simulink model "CHEM_FULL_BENCHMARK"  (R2019a)
settings: Solver=FixedStepAuto  StartTime=0.0  StopTime=app.SimuTime  FixedStep=Te  RelTol=1e-3  EnableMultiTasking=on
values from neighbouring files (symbols this model uses):
  A1 = 0.0154    [INIT_FULL.m]    (also in run.m)
  A2 = 0.0154    [INIT_FULL.m]    (also in run.m)
  app = interface    [INIT_FULL.m]    (also in run.m)
  Cvb = 1.5938*1e-4    (= 0.00015938)    [INIT_FULL.m]    (also in run.m)
  Cvo = 1.59640*1e-4    (= 0.00015964)    [INIT_FULL.m]    (also in run.m)
  g = 9.81    [INIT_FULL.m]    (also in run.m)
  h1c = 0.5    [INIT_FULL.m]    (also in run.m)
  h1c_0 = 0    [INIT_FULL.m]    (also in run.m)
  h1max = 0.6    [INIT_FULL.m]    (also in run.m)
  h2c_0 = 0    [INIT_FULL.m]    (also in Variables_Update.m = app.InitialwaterlevelinT206EditField.Value; run.m)
  h2c_max = 0.11    [INIT_FULL.m]    (also in run.m)
  h2c_min = 0.09    [INIT_FULL.m]    (also in run.m)
  h2max = 0.6    [INIT_FULL.m]    (also in run.m)
  Ki = 5*1e-6    (= 5e-06)    [INIT_FULL.m]    (also in run.m)
  Kp = 1e-3    (= 0.001)    [INIT_FULL.m]    (also in run.m)
  Patm = 101325    [INIT_FULL.m]    (also in run.m)
  Qf1 = 1e-4    (= 0.0001)    [INIT_FULL.m]    (also in Variables_Update.m = app.FlowleakfromT1m3sEditField.Value; run.m)
  Qf2 = 1e-4    (= 0.0001)    [INIT_FULL.m]    (also in Variables_Update.m = app.FlowleakfromT2m3sEditField.Value; run.m)
  Qof1 = 1e-4    (= 0.0001)    [INIT_FULL.m]    (also in Variables_Update.m = app.OverflowrateinT1m3sEditField.Value; run.m)
  Qpmax = 1e-2    (= 0.01)    [INIT_FULL.m]    (also in run.m)
  rate_noise_mQp = 0.01*1e-5    (= 1e-07)    [INIT_FULL.m]    (also in run.m)
  rate_noise_mUp = 0.01*1e-5    (= 1e-07)    [INIT_FULL.m]    (also in run.m)
  rate_noise_my1 = 0.5*0.001    (= 0.0005)    [INIT_FULL.m]    (also in run.m)
  rate_noise_my2 = 0.3*0.001    (= 0.0003)    [INIT_FULL.m]    (also in run.m)
  ro = 1000    [INIT_FULL.m]    (also in run.m)
  seed = randi(10000000)    [INIT_FULL.m]    (also in run.m)
  Te = 1    [INIT_FULL.m]    (also in run.m)
  yo = 0    [INIT_FULL.m]    (also in run.m)
(part 1 of 12)
settings Model: Creator=upcnet  LastModifiedBy=etse
settings DataIOCC: LimitDataPoints=on  SaveFormat=Array  ReturnWorkspaceOutputs=off  SignalLoggingName=sigsOut
settings OptimizationCC: BlockReduction=off  BooleanDataType=off  LifeSpan=inf
settings DebuggingCC: AlgebraicLoopMsg=none  SaveWithParameterizedLinksMsg=none  UnderspecifiedInitializationDetection=Classic  MergeDetectMultiDrivingBlocksExec=none  SignalResolutionControl=TryResolveAllWithWarning  MultiTaskDSMMsg=warning  MultiTaskCondExecSysMsg=none  AllowSymbolicDim=off  PregeneratedLibrarySubsystemCodeDiagnostic=none  SFUnexpectedBacktrackingDiag=warning  SFNoUnconditionalDefaultTransitionDiag=warning  SFExecutionAtInitializationDiag=none  ArithmeticOperatorsInVariantConditions=warning
settings HardwareCC: ProdBitPerPointer=32  ProdBitPerSizeT=32  ProdBitPerPtrDiffT=32  ProdLargestAtomicFloat=None  ProdIntDivRoundTo=Undefined  ProdEndianess=Unspecified  ProdWordSize=32  ProdHWDeviceType=32-bit Generic  TargetUnknown=on
settings ModelReferenceCC: PropagateSignalLabelsOutOfModel=off
settings SFSimCC: SimUseLocalCustomCode=off
settings RTWCC: RTWUseLocalCustomCode=off
settings CodeAppCC: StateflowObjectComments=on
settings GRTTargetCC: TargetLangStandard=C89/C90 (ANSI)  CombineOutputUpdateFcns=off  GRTInterface=on
settings ConfigComp: CovMetricSettings=dw  CovHtmlReporting=on  CovSaveCumulativeToWorkspaceVar=on  CovSaveSingleToWorkspaceVar=on  CovExternalEMLEnable=off

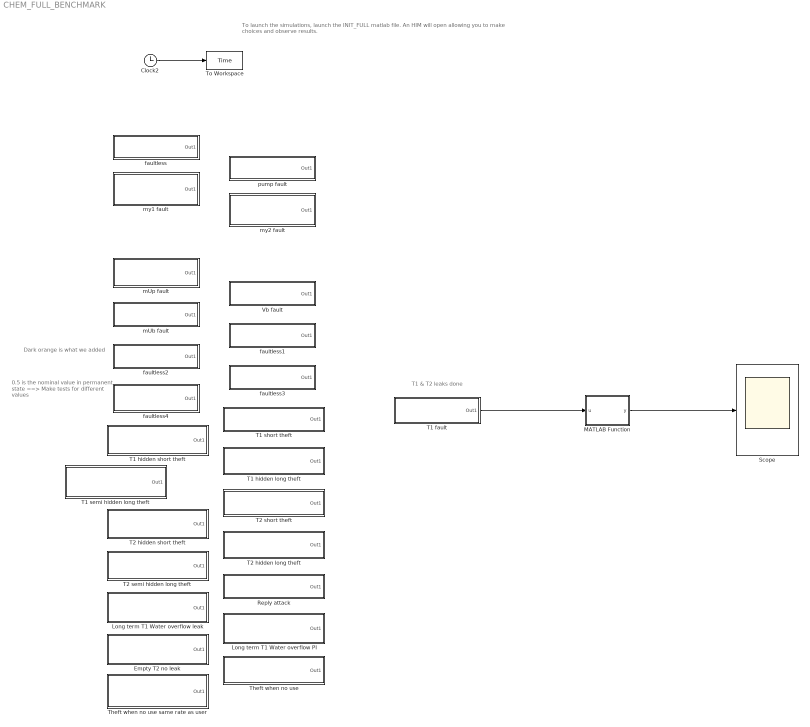
== system CHEM_FULL_BENCHMARK ==
  note: T1 & T2 leaks done
  note: To launch the simulations, launch the INIT_FULL matlab file. An HIM will open allowing you to make choices and observe results.
  note: 0.5 is the nominal value
      | in permanent  state
      | ==> Make tests for different values
  note: Dark orange is what we added
  Clock2 : Clock
  Empty T2 no leak : Subsystem
      mask Display: disp('25) Attack 12\nEmptying T2 without leak')
  Long term T1 Water overflow PI : Subsystem
      mask Display: disp('24) Attack 11\nLong term T1 Water overflow\nWith PI pass by')
  Long term T1 Water overflow leak : Subsystem
      mask Display: disp('23) Attack 10\nLong term T1 Water overflow\nWith simulated leak')
  MATLAB Function : MATLAB Function  TreatAsAtomicUnit=on
  Reply attack : Subsystem
      mask Display: disp('22) Attack 9\nReplay attack')
  Scope : Scope
  T1 fault : Subsystem
      mask Display: disp('5) Fault 4\nTank T1 leak fault: Qf1')
  T1 hidden long theft : Subsystem
      mask Display: disp('16) Attack 3\nLong-term water theft of T1\n without any change of my1')
  T1 hidden short theft : Subsystem
      mask Display: disp('15) Attack 2\nShort-term water theft of T1\n without any change of my1')
  T1 semi hidden long theft : Subsystem
      mask Display: disp('17) Attack 4\nLong-term water theft of T1\nwith a small change of my1')
  T1 short theft : Subsystem
      mask Display: disp('14) Attack 1\nShort-term water theft of T1')
  T2 hidden long theft : Subsystem
      mask Display: disp('20) Attack 7\nLong-term water theft of T2\n without any change of my2')
  T2 hidden short theft : Subsystem
      mask Display: disp('19) Attack 6\nShort-term water theft of T2\n without any change of my2')
  T2 semi hidden long theft : Subsystem
      mask Display: disp('21) Attack 8\nLong-term water theft of T2\n with a small change of my2')
  T2 short theft : Subsystem
      mask Display: disp('18) Attack 5\nShort-term water theft of T2')
  Theft when no use : Subsystem
      mask Display: disp('26) Attack 13\nTheft in T2 when user is not\npumping water')
  Theft when no use same rate as user : Subsystem
      mask Display: disp('27) Attack 14\nTheft in T2 when user is not\npumping water, at the same\nrate as user')
  To Workspace : ToWorkspace  VariableName=Time  SampleTime=-1
  Vb fault : Subsystem
      mask Display: disp('8) Fault 7\nValve Vb stuck closed')
  faultless : Subsystem
      mask Display: disp('1)\nNominal mode')
  faultless1 : Subsystem
      mask Display: disp('10) Fault 9\nSensor fault Qp')
  faultless2 : Subsystem
      mask Display: disp('11) Fault 10\nPI controller KO')
  faultless3 : Subsystem
      mask Display: disp('12) Fault 11\nValve Vb stuck open')
  faultless4 : Subsystem
      mask Display: disp('13) Fault 12\nSensor T1 default\ndifferent from 0')
  mUb fault : Subsystem
      mask Display: disp('9) Fault 8\nSensor fault mUb')
  mUp fault : Subsystem
      mask Display: disp('7) Fault 6\nSensor fault mUp')
  my1 fault : Subsystem
      mask Display: disp('3) Fault 2\nLevel sensor fault\n of tank T1: my1')
  my2 fault : Subsystem
      mask Display: disp('4) Fault 3\nLevel sensor fault\n of tank T2: my2')
  pump fault : Subsystem
      mask Display: disp('2) Fault 1\nPump fault')
  wires:
  Clock2/1 -> To Workspace/1
  MATLAB Function/1(y) -> Scope/1
  T1 fault/1(Out1) -> MATLAB Function/1(u)

== system CHEM_FULL_BENCHMARK/Empty T2 no leak ==
  note: mP2
  note: mP1
  note: mUp
  note: mQp
  note: Uo
  note: y1
  note: y2
  note: h1c
  note: mUb
  note: vol2
  note: my1
  note: mQ0
  note: my2
  note: vol1
  Mux : Mux  Inputs=14
  Process : Subsystem
      mask Display: disp('P\nR\nO\nC\nE\nS\nS')
  Out1 : Outport
  wires:
  Process/14(mP2) -> Mux/14
  Process/13(mP1) -> Mux/13
  Process/8(mq0) -> Mux/8
  Process/5(my2) -> Mux/5
  Process/10(vol1) -> Mux/10
  Process/3("Uo ") -> Mux/3
  Process/2(mUb) -> Mux/2
  Process/1(mQp) -> Mux/1
  Process/4(my1) -> Mux/4
  Process/11(y2) -> Mux/11
  Mux/1 -> Out1/1
  Process/6(h1c) -> Mux/6
  Process/9(y1) -> Mux/9
  Process/12(vol2) -> Mux/12
  Process/7(mUp) -> Mux/7

== system CHEM_FULL_BENCHMARK/Long term T1 Water overflow PI ==
  note: mP2
  note: mP1
  note: mUp
  note: mQp
  note: Uo
  note: y1
  note: y2
  note: h1c
  note: mUb
  note: vol2
  note: my1
  note: mQ0
  note: my2
  note: vol1
  Mux : Mux  Inputs=14
  Process : Subsystem
      mask Display: disp('P\nR\nO\nC\nE\nS\nS')
  Out1 : Outport
  wires:
  Process/14(mP2) -> Mux/14
  Process/13(mP1) -> Mux/13
  Process/8(mq0) -> Mux/8
  Process/5(my2) -> Mux/5
  Process/10(vol1) -> Mux/10
  Process/3("Uo ") -> Mux/3
  Process/2(mUb) -> Mux/2
  Process/1(mQp) -> Mux/1
  Process/4(my1) -> Mux/4
  Process/11(y2) -> Mux/11
  Mux/1 -> Out1/1
  Process/6(h1c) -> Mux/6
  Process/9(y1) -> Mux/9
  Process/12(vol2) -> Mux/12
  Process/7(mUp) -> Mux/7

== system CHEM_FULL_BENCHMARK/Long term T1 Water overflow leak ==
  note: mP2
  note: mP1
  note: mUp
  note: mQp
  note: Uo
  note: y1
  note: y2
  note: h1c
  note: mUb
  note: vol2
  note: my1
  note: mQ0
  note: my2
  note: vol1
  Mux : Mux  Inputs=14
  Process : Subsystem
      mask Display: disp('P\nR\nO\nC\nE\nS\nS')
  Out1 : Outport
  wires:
  Process/14(mP2) -> Mux/14
  Process/13(mP1) -> Mux/13
  Process/8(mq0) -> Mux/8
  Process/5(my2) -> Mux/5
  Process/10(vol1) -> Mux/10
  Process/3("Uo ") -> Mux/3
  Process/2(mUb) -> Mux/2
  Process/1(mQp) -> Mux/1
  Process/4(my1) -> Mux/4
  Process/11(y2) -> Mux/11
  Mux/1 -> Out1/1
  Process/6(h1c) -> Mux/6
  Process/9(y1) -> Mux/9
  Process/12(vol2) -> Mux/12
  Process/7(mUp) -> Mux/7

== system CHEM_FULL_BENCHMARK/Reply attack ==
  note: mP2
  note: mP1
  note: mUp
  note: mQp
  note: Uo
  note: y1
  note: y2
  note: h1c
  note: mUb
  note: vol2
  note: my1
  note: mQ0
  note: my2
  note: vol1
  Mux : Mux  Inputs=14
  Process : Subsystem
      mask Display: disp('P\nR\nO\nC\nE\nS\nS')
  Out1 : Outport
  wires:
  Process/14(mP2) -> Mux/14
  Process/13(mP1) -> Mux/13
  Process/8(mq0) -> Mux/8
  Process/5(my2) -> Mux/5
  Process/10(vol1) -> Mux/10
  Process/3("Uo ") -> Mux/3
  Process/2(mUb) -> Mux/2
  Process/1(mQp) -> Mux/1
  Process/4(my1) -> Mux/4
  Process/11(y2) -> Mux/11
  Mux/1 -> Out1/1
  Process/6(h1c) -> Mux/6
  Process/9(y1) -> Mux/9
  Process/12(vol2) -> Mux/12
  Process/7(mUp) -> Mux/7

== system CHEM_FULL_BENCHMARK/T1 fault ==
  note: mP2
  note: mP1
  note: mUp
  note: mQp
  note: Uo
  note: y1
  note: y2
  note: h1c
  note: mUb
  note: vol2
  note: my1
  note: mQ0
  note: my2
  note: vol1
  Mux : Mux  Inputs=14
  Process : Subsystem
      mask Display: disp('P\nR\nO\nC\nE\nS\nS')
  Out1 : Outport
  wires:
  Process/14(mP2) -> Mux/14
  Process/13(mP1) -> Mux/13
  Process/8(mq0) -> Mux/8
  Process/5(my2) -> Mux/5
  Process/10(vol1) -> Mux/10
  Process/3("Uo ") -> Mux/3
  Process/2(mUb) -> Mux/2
  Process/1(mQp) -> Mux/1
  Process/4(my1) -> Mux/4
  Process/11(y2) -> Mux/11
  Mux/1 -> Out1/1
  Process/6(h1c) -> Mux/6
  Process/9(y1) -> Mux/9
  Process/12(vol2) -> Mux/12
  Process/7(mUp) -> Mux/7

== system CHEM_FULL_BENCHMARK/T1 hidden long theft ==
  note: mP2
  note: mP1
  note: mUp
  note: mQp
  note: Uo
  note: y1
  note: y2
  note: h1c
  note: mUb
  note: vol2
  note: my1
  note: mQ0
  note: my2
  note: vol1
  Mux : Mux  Inputs=14
  Process : Subsystem
      mask Display: disp('P\nR\nO\nC\nE\nS\nS')
  Out1 : Outport
  wires:
  Process/14(mP2) -> Mux/14
  Process/13(mP1) -> Mux/13
  Process/8(mq0) -> Mux/8
  Process/5(my2) -> Mux/5
  Process/10(vol1) -> Mux/10
  Process/3("Uo ") -> Mux/3
  Process/2(mUb) -> Mux/2
  Process/1(mQp) -> Mux/1
  Process/4(my1) -> Mux/4
  Process/11(y2) -> Mux/11
  Mux/1 -> Out1/1
  Process/6(h1c) -> Mux/6
  Process/9(y1) -> Mux/9
  Process/12(vol2) -> Mux/12
  Process/7(mUp) -> Mux/7

== system CHEM_FULL_BENCHMARK/T1 hidden short theft ==
  note: mP2
  note: mP1
  note: mUp
  note: mQp
  note: Uo
  note: y1
  note: y2
  note: h1c
  note: mUb
  note: vol2
  note: my1
  note: mQ0
  note: my2
  note: vol1
  Mux : Mux  Inputs=14
  Process : Subsystem
      mask Display: disp('P\nR\nO\nC\nE\nS\nS')
  Out1 : Outport
  wires:
  Process/14(mP2) -> Mux/14
  Process/13(mP1) -> Mux/13
  Process/8(mq0) -> Mux/8
  Process/5(my2) -> Mux/5
  Process/10(vol1) -> Mux/10
  Process/3("Uo ") -> Mux/3
  Process/2(mUb) -> Mux/2
  Process/1(mQp) -> Mux/1
  Process/4(my1) -> Mux/4
  Process/11(y2) -> Mux/11
  Mux/1 -> Out1/1
  Process/6(h1c) -> Mux/6
  Process/9(y1) -> Mux/9
  Process/12(vol2) -> Mux/12
  Process/7(mUp) -> Mux/7

== system CHEM_FULL_BENCHMARK/T1 semi hidden long theft ==
  note: mP2
  note: mP1
  note: mUp
  note: mQp
  note: Uo
  note: y1
  note: y2
  note: h1c
  note: mUb
  note: vol2
  note: my1
  note: mQ0
  note: my2
  note: vol1
  Mux : Mux  Inputs=14
  Process : Subsystem
      mask Display: disp('P\nR\nO\nC\nE\nS\nS')
  Out1 : Outport
  wires:
  Process/14(mP2) -> Mux/14
  Process/13(mP1) -> Mux/13
  Process/8(mq0) -> Mux/8
  Process/5(my2) -> Mux/5
  Process/10(vol1) -> Mux/10
  Process/3("Uo ") -> Mux/3
  Process/2(mUb) -> Mux/2
  Process/1(mQp) -> Mux/1
  Process/4(my1) -> Mux/4
  Process/11(y2) -> Mux/11
  Mux/1 -> Out1/1
  Process/6(h1c) -> Mux/6
  Process/9(y1) -> Mux/9
  Process/12(vol2) -> Mux/12
  Process/7(mUp) -> Mux/7

== system CHEM_FULL_BENCHMARK/T1 short theft ==
  note: mP2
  note: mP1
  note: mUp
  note: mQp
  note: Uo
  note: y1
  note: y2
  note: h1c
  note: mUb
  note: vol2
  note: my1
  note: mQ0
  note: my2
  note: vol1
  Mux : Mux  Inputs=14
  Process : Subsystem
      mask Display: disp('P\nR\nO\nC\nE\nS\nS')
  Out1 : Outport
  wires:
  Process/14(mP2) -> Mux/14
  Process/13(mP1) -> Mux/13
  Process/8(mq0) -> Mux/8
  Process/5(my2) -> Mux/5
  Process/10(vol1) -> Mux/10
  Process/3("Uo ") -> Mux/3
  Process/2(mUb) -> Mux/2
  Process/1(mQp) -> Mux/1
  Process/4(my1) -> Mux/4
  Process/11(y2) -> Mux/11
  Mux/1 -> Out1/1
  Process/6(h1c) -> Mux/6
  Process/9(y1) -> Mux/9
  Process/12(vol2) -> Mux/12
  Process/7(mUp) -> Mux/7

== system CHEM_FULL_BENCHMARK/T2 hidden long theft ==
  note: mP2
  note: mP1
  note: mUp
  note: mQp
  note: Uo
  note: y1
  note: y2
  note: h1c
  note: mUb
  note: vol2
  note: my1
  note: mQ0
  note: my2
  note: vol1
  Mux : Mux  Inputs=14
  Process : Subsystem
      mask Display: disp('P\nR\nO\nC\nE\nS\nS')
  Out1 : Outport
  wires:
  Process/14(mP2) -> Mux/14
  Process/13(mP1) -> Mux/13
  Process/8(mq0) -> Mux/8
  Process/5(my2) -> Mux/5
  Process/10(vol1) -> Mux/10
  Process/3("Uo ") -> Mux/3
  Process/2(mUb) -> Mux/2
  Process/1(mQp) -> Mux/1
  Process/4(my1) -> Mux/4
  Process/11(y2) -> Mux/11
  Mux/1 -> Out1/1
  Process/6(h1c) -> Mux/6
  Process/9(y1) -> Mux/9
  Process/12(vol2) -> Mux/12
  Process/7(mUp) -> Mux/7

== system CHEM_FULL_BENCHMARK/T2 hidden short theft ==
  note: mP2
  note: mP1
  note: mUp
  note: mQp
  note: Uo
  note: y1
  note: y2
  note: h1c
  note: mUb
  note: vol2
  note: my1
  note: mQ0
  note: my2
  note: vol1
  Mux : Mux  Inputs=14
  Process : Subsystem
      mask Display: disp('P\nR\nO\nC\nE\nS\nS')
  Out1 : Outport
  wires:
  Process/14(mP2) -> Mux/14
  Process/13(mP1) -> Mux/13
  Process/8(mq0) -> Mux/8
  Process/5(my2) -> Mux/5
  Process/10(vol1) -> Mux/10
  Process/3("Uo ") -> Mux/3
  Process/2(mUb) -> Mux/2
  Process/1(mQp) -> Mux/1
  Process/4(my1) -> Mux/4
  Process/11(y2) -> Mux/11
  Mux/1 -> Out1/1
  Process/6(h1c) -> Mux/6
  Process/9(y1) -> Mux/9
  Process/12(vol2) -> Mux/12
  Process/7(mUp) -> Mux/7

== system CHEM_FULL_BENCHMARK/T2 semi hidden long theft ==
  note: mP2
  note: mP1
  note: mUp
  note: mQp
  note: Uo
  note: y1
  note: y2
  note: h1c
  note: mUb
  note: vol2
  note: my1
  note: mQ0
  note: my2
  note: vol1
  Mux : Mux  Inputs=14
  Process : Subsystem
      mask Display: disp('P\nR\nO\nC\nE\nS\nS')
  Out1 : Outport
  wires:
  Process/14(mP2) -> Mux/14
  Process/13(mP1) -> Mux/13
  Process/8(mq0) -> Mux/8
  Process/5(my2) -> Mux/5
  Process/10(vol1) -> Mux/10
  Process/3("Uo ") -> Mux/3
  Process/2(mUb) -> Mux/2
  Process/1(mQp) -> Mux/1
  Process/4(my1) -> Mux/4
  Process/11(y2) -> Mux/11
  Mux/1 -> Out1/1
  Process/6(h1c) -> Mux/6
  Process/9(y1) -> Mux/9
  Process/12(vol2) -> Mux/12
  Process/7(mUp) -> Mux/7

== system CHEM_FULL_BENCHMARK/T2 short theft ==
  note: mP2
  note: mP1
  note: mUp
  note: mQp
  note: Uo
  note: y1
  note: y2
  note: h1c
  note: mUb
  note: vol2
  note: my1
  note: mQ0
  note: my2
  note: vol1
  Mux : Mux  Inputs=14
  Process : Subsystem
      mask Display: disp('P\nR\nO\nC\nE\nS\nS')
  Out1 : Outport
  wires:
  Process/14(mP2) -> Mux/14
  Process/13(mP1) -> Mux/13
  Process/8(mq0) -> Mux/8
  Process/5(my2) -> Mux/5
  Process/10(vol1) -> Mux/10
  Process/3("Uo ") -> Mux/3
  Process/2(mUb) -> Mux/2
  Process/1(mQp) -> Mux/1
  Process/4(my1) -> Mux/4
  Process/11(y2) -> Mux/11
  Mux/1 -> Out1/1
  Process/6(h1c) -> Mux/6
  Process/9(y1) -> Mux/9
  Process/12(vol2) -> Mux/12
  Process/7(mUp) -> Mux/7

== system CHEM_FULL_BENCHMARK/Theft when no use ==
  note: mP2
  note: mP1
  note: mUp
  note: mQp
  note: Uo
  note: y1
  note: y2
  note: h1c
  note: mUb
  note: vol2
  note: my1
  note: mQ0
  note: my2
  note: vol1
  Mux : Mux  Inputs=14
  Process : Subsystem
      mask Display: disp('P\nR\nO\nC\nE\nS\nS')
  Out1 : Outport
  wires:
  Process/14(mP2) -> Mux/14
  Process/13(mP1) -> Mux/13
  Process/8(mq0) -> Mux/8
  Process/5(my2) -> Mux/5
  Process/10(vol1) -> Mux/10
  Process/3("Uo ") -> Mux/3
  Process/2(mUb) -> Mux/2
  Process/1(mQp) -> Mux/1
  Process/4(my1) -> Mux/4
  Process/11(y2) -> Mux/11
  Mux/1 -> Out1/1
  Process/6(h1c) -> Mux/6
  Process/9(y1) -> Mux/9
  Process/12(vol2) -> Mux/12
  Process/7(mUp) -> Mux/7

== system CHEM_FULL_BENCHMARK/Theft when no use same rate as user ==
  note: mP2
  note: mP1
  note: mUp
  note: mQp
  note: Uo
  note: y1
  note: y2
  note: h1c
  note: mUb
  note: vol2
  note: my1
  note: mQ0
  note: my2
  note: vol1
  Mux : Mux  Inputs=14
  Process : Subsystem
      mask Display: disp('P\nR\nO\nC\nE\nS\nS')
  Out1 : Outport
  wires:
  Process/14(mP2) -> Mux/14
  Process/13(mP1) -> Mux/13
  Process/8(mq0) -> Mux/8
  Process/5(my2) -> Mux/5
  Process/10(vol1) -> Mux/10
  Process/3("Uo ") -> Mux/3
  Process/2(mUb) -> Mux/2
  Process/1(mQp) -> Mux/1
  Process/4(my1) -> Mux/4
  Process/11(y2) -> Mux/11
  Mux/1 -> Out1/1
  Process/6(h1c) -> Mux/6
  Process/9(y1) -> Mux/9
  Process/12(vol2) -> Mux/12
  Process/7(mUp) -> Mux/7

== system CHEM_FULL_BENCHMARK/Vb fault ==
  note: mP2
  note: mP1
  note: mUp
  note: mQp
  note: Uo
  note: y1
  note: y2
  note: h1c
  note: mUb
  note: vol2
  note: my1
  note: mQ0
  note: my2
  note: vol1
  Mux : Mux  Inputs=14
  Process : Subsystem
      mask Display: disp('P\nR\nO\nC\nE\nS\nS')
  Out1 : Outport
  wires:
  Process/14(mP2) -> Mux/14
  Process/13(mP1) -> Mux/13
  Process/8(mq0) -> Mux/8
  Process/5(my2) -> Mux/5
  Process/10(vol1) -> Mux/10
  Process/3("Uo ") -> Mux/3
  Process/2(mUb) -> Mux/2
  Process/1(mQp) -> Mux/1
  Process/4(my1) -> Mux/4
  Process/11(y2) -> Mux/11
  Mux/1 -> Out1/1
  Process/6(h1c) -> Mux/6
  Process/9(y1) -> Mux/9
  Process/12(vol2) -> Mux/12
  Process/7(mUp) -> Mux/7

== system CHEM_FULL_BENCHMARK/faultless ==
  note: my2
  note: vol1
  note: mUp
  note: Uo
  note: my1
  note: mQ0
  note: mQp
  note: y1
  note: mUb
  note: y2
  note: h1c
  note: vol2
  note: mP1
  note: mP2
  Mux : Mux  Inputs=14
  Process : Subsystem
      mask Display: disp('P\nR\nO\nC\nE\nS\nS')
  Out1 : Outport
  wires:
  Process/5(my2) -> Mux/5
  Process/1(mQp) -> Mux/1
  Process/9(y1) -> Mux/9
  Process/6(h1c) -> Mux/6
  Mux/1 -> Out1/1
  Process/2(mUb) -> Mux/2
  Process/7(mUp) -> Mux/7
  Process/11(y2) -> Mux/11
  Process/10(vol1) -> Mux/10
  Process/3("Uo ") -> Mux/3
  Process/4(my1) -> Mux/4
  Process/12(vol2) -> Mux/12
  Process/8(mq0) -> Mux/8
  Process/13(mP1) -> Mux/13
  Process/14(mP2) -> Mux/14

== system CHEM_FULL_BENCHMARK/faultless1 ==
  note: mP2
  note: mP1
  note: mUp
  note: mQp
  note: Uo
  note: y1
  note: y2
  note: h1c
  note: mUb
  note: vol2
  note: my1
  note: mQ0
  note: my2
  note: vol1
  Mux : Mux  Inputs=14
  Process : Subsystem
      mask Display: disp('P\nR\nO\nC\nE\nS\nS')
  Out1 : Outport
  wires:
  Process/14(mP2) -> Mux/14
  Process/13(mP1) -> Mux/13
  Process/8(mq0) -> Mux/8
  Process/5(my2) -> Mux/5
  Process/10(vol1) -> Mux/10
  Process/3("Uo ") -> Mux/3
  Process/2(mUb) -> Mux/2
  Process/1(mQp) -> Mux/1
  Process/4(my1) -> Mux/4
  Process/11(y2) -> Mux/11
  Mux/1 -> Out1/1
  Process/6(h1c) -> Mux/6
  Process/9(y1) -> Mux/9
  Process/12(vol2) -> Mux/12
  Process/7(mUp) -> Mux/7

== system CHEM_FULL_BENCHMARK/faultless2 ==
  note: mP2
  note: mP1
  note: mUp
  note: mQp
  note: Uo
  note: y1
  note: y2
  note: h1c
  note: mUb
  note: vol2
  note: my1
  note: mQ0
  note: my2
  note: vol1
  Mux : Mux  Inputs=14
  Process : Subsystem
      mask Display: disp('P\nR\nO\nC\nE\nS\nS')
  Out1 : Outport
  wires:
  Process/14(mP2) -> Mux/14
  Process/13(mP1) -> Mux/13
  Process/8(mq0) -> Mux/8
  Process/5(my2) -> Mux/5
  Process/10(vol1) -> Mux/10
  Process/3("Uo ") -> Mux/3
  Process/2(mUb) -> Mux/2
  Process/1(mQp) -> Mux/1
  Process/4(my1) -> Mux/4
  Process/11(y2) -> Mux/11
  Mux/1 -> Out1/1
  Process/6(h1c) -> Mux/6
  Process/9(y1) -> Mux/9
  Process/12(vol2) -> Mux/12
  Process/7(mUp) -> Mux/7

== system CHEM_FULL_BENCHMARK/faultless3 ==
  note: mP2
  note: mP1
  note: mUp
  note: mQp
  note: Uo
  note: y1
  note: y2
  note: h1c
  note: mUb
  note: vol2
  note: my1
  note: mQ0
  note: my2
  note: vol1
  Mux : Mux  Inputs=14
  Process : Subsystem
      mask Display: disp('P\nR\nO\nC\nE\nS\nS')
  Out1 : Outport
  wires:
  Process/14(mP2) -> Mux/14
  Process/13(mP1) -> Mux/13
  Process/8(mq0) -> Mux/8
  Process/5(my2) -> Mux/5
  Process/10(vol1) -> Mux/10
  Process/3("Uo ") -> Mux/3
  Process/2(mUb) -> Mux/2
  Process/1(mQp) -> Mux/1
  Process/4(my1) -> Mux/4
  Process/11(y2) -> Mux/11
  Mux/1 -> Out1/1
  Process/6(h1c) -> Mux/6
  Process/9(y1) -> Mux/9
  Process/12(vol2) -> Mux/12
  Process/7(mUp) -> Mux/7

== system CHEM_FULL_BENCHMARK/faultless4 ==
  note: mP2
  note: mP1
  note: mUp
  note: mQp
  note: Uo
  note: y1
  note: y2
  note: h1c
  note: mUb
  note: vol2
  note: my1
  note: mQ0
  note: my2
  note: vol1
  Mux : Mux  Inputs=14
  Process : Subsystem
      mask Display: disp('P\nR\nO\nC\nE\nS\nS')
  Out1 : Outport
  wires:
  Process/14(mP2) -> Mux/14
  Process/13(mP1) -> Mux/13
  Process/8(mq0) -> Mux/8
  Process/5(my2) -> Mux/5
  Process/10(vol1) -> Mux/10
  Process/3("Uo ") -> Mux/3
  Process/2(mUb) -> Mux/2
  Process/1(mQp) -> Mux/1
  Process/4(my1) -> Mux/4
  Process/11(y2) -> Mux/11
  Mux/1 -> Out1/1
  Process/6(h1c) -> Mux/6
  Process/9(y1) -> Mux/9
  Process/12(vol2) -> Mux/12
  Process/7(mUp) -> Mux/7

== system CHEM_FULL_BENCHMARK/mUb fault ==
  note: mP2
  note: mP1
  note: mUp
  note: mQp
  note: Uo
  note: y1
  note: y2
  note: h1c
  note: mUb
  note: vol2
  note: my1
  note: mQ0
  note: my2
  note: vol1
  Mux : Mux  Inputs=14
  Process : Subsystem
      mask Display: disp('P\nR\nO\nC\nE\nS\nS')
  Out1 : Outport
  wires:
  Process/14(mP2) -> Mux/14
  Process/13(mP1) -> Mux/13
  Process/8(mq0) -> Mux/8
  Process/5(my2) -> Mux/5
  Process/10(vol1) -> Mux/10
  Process/3("Uo ") -> Mux/3
  Process/2(mUb) -> Mux/2
  Process/1(mQp) -> Mux/1
  Process/4(my1) -> Mux/4
  Process/11(y2) -> Mux/11
  Mux/1 -> Out1/1
  Process/6(h1c) -> Mux/6
  Process/9(y1) -> Mux/9
  Process/12(vol2) -> Mux/12
  Process/7(mUp) -> Mux/7

== system CHEM_FULL_BENCHMARK/mUp fault ==
  note: mP2
  note: mP1
  note: mUp
  note: mQp
  note: Uo
  note: y1
  note: y2
  note: h1c
  note: mUb
  note: vol2
  note: my1
  note: mQ0
  note: my2
  note: vol1
  Mux : Mux  Inputs=14
  Process : Subsystem
      mask Display: disp('P\nR\nO\nC\nE\nS\nS')
  Out1 : Outport
  wires:
  Process/14(mP2) -> Mux/14
  Process/13(mP1) -> Mux/13
  Process/8(mq0) -> Mux/8
  Process/5(my2) -> Mux/5
  Process/10(vol1) -> Mux/10
  Process/3("Uo ") -> Mux/3
  Process/2(mUb) -> Mux/2
  Process/1(mQp) -> Mux/1
  Process/4(my1) -> Mux/4
  Process/11(y2) -> Mux/11
  Mux/1 -> Out1/1
  Process/6(h1c) -> Mux/6
  Process/9(y1) -> Mux/9
  Process/12(vol2) -> Mux/12
  Process/7(mUp) -> Mux/7

== system CHEM_FULL_BENCHMARK/my1 fault ==
  note: mP2
  note: mP1
  note: mUp
  note: mQp
  note: Uo
  note: y1
  note: y2
  note: h1c
  note: mUb
  note: vol2
  note: my1
  note: mQ0
  note: my2
  note: vol1
  Mux : Mux  Inputs=14
  Process : Subsystem
      mask Display: disp('P\nR\nO\nC\nE\nS\nS')
  Out1 : Outport
  wires:
  Process/14(mP2) -> Mux/14
  Process/13(mP1) -> Mux/13
  Process/8(mq0) -> Mux/8
  Process/5(my2) -> Mux/5
  Process/10(vol1) -> Mux/10
  Process/3("Uo ") -> Mux/3
  Process/2(mUb) -> Mux/2
  Process/1(mQp) -> Mux/1
  Process/4(my1) -> Mux/4
  Process/11(y2) -> Mux/11
  Mux/1 -> Out1/1
  Process/6(h1c) -> Mux/6
  Process/9(y1) -> Mux/9
  Process/12(vol2) -> Mux/12
  Process/7(mUp) -> Mux/7

== system CHEM_FULL_BENCHMARK/my2 fault ==
  note: mP2
  note: mP1
  note: mUp
  note: mQp
  note: Uo
  note: y1
  note: y2
  note: h1c
  note: mUb
  note: vol2
  note: my1
  note: mQ0
  note: my2
  note: vol1
  Mux : Mux  Inputs=14
  Process : Subsystem
      mask Display: disp('P\nR\nO\nC\nE\nS\nS')
  Out1 : Outport
  wires:
  Process/14(mP2) -> Mux/14
  Process/13(mP1) -> Mux/13
  Process/8(mq0) -> Mux/8
  Process/5(my2) -> Mux/5
  Process/10(vol1) -> Mux/10
  Process/3("Uo ") -> Mux/3
  Process/2(mUb) -> Mux/2
  Process/1(mQp) -> Mux/1
  Process/4(my1) -> Mux/4
  Process/11(y2) -> Mux/11
  Mux/1 -> Out1/1
  Process/6(h1c) -> Mux/6
  Process/9(y1) -> Mux/9
  Process/12(vol2) -> Mux/12
  Process/7(mUp) -> Mux/7

== system CHEM_FULL_BENCHMARK/pump fault ==
  note: mUb
  note: y2
  note: mQp
  note: my2
  note: mUp
  note: Uo
  note: y1
  note: mQ0
  note: h1c
  note: vol1
  note: vol2
  note: my1
  note: mP1
  note: mP2
  Mux : Mux  Inputs=14
  Process : Subsystem
      mask Display: disp('P\nR\nO\nC\nE\nS\nS')
  Out1 : Outport
  wires:
  Process/4(my1) -> Mux/4
  Process/3("Uo ") -> Mux/3
  Process/12(vol2) -> Mux/12
  Process/2(mUb) -> Mux/2
  Mux/1 -> Out1/1
  Process/9(y1) -> Mux/9
  Process/6(h1c) -> Mux/6
  Process/11(y2) -> Mux/11
  Process/7(mUp) -> Mux/7
  Process/10(vol1) -> Mux/10
  Process/5(my2) -> Mux/5
  Process/1(mQp) -> Mux/1
  Process/8(mq0) -> Mux/8
  Process/13(mP1) -> Mux/13
  Process/14(mP2) -> Mux/14

== system CHEM_FULL_BENCHMARK/Empty T2 no leak/Process ==
  note: y2
  note: y1
  note: Ub
  note: Up
  note: Qvo
      | To users
  note: Qp
  note: Qvb
  Constant : Constant  Value=yo
  Subsystem1 : Subsystem
      mask Display: disp('TANK 1')
  Subsystem10 : Subsystem
      mask Display: disp('Sensor\n y2')
  Subsystem11 : Subsystem
      mask Display: disp('Controller 1')
  Subsystem12 : Subsystem
      mask Display: disp('Sensor\n Ub')
  Subsystem13 : Subsystem
      mask Display: disp('Sensor\n Up')
  Subsystem14 : Subsystem
      mask Display: disp('Sensor\n Qp')
  Subsystem15 : Subsystem
      mask Display: disp('Sensor\n P2')
  Subsystem2 : Subsystem
      mask Display: disp('Valve B')
  Subsystem3 : Subsystem
      mask Display: disp('Valve O')
  Subsystem4 : Subsystem
      mask Display: disp('Controller2')
  Subsystem5 : Subsystem
      mask Display: disp('Sensor\n P1')
  Subsystem6 : Subsystem
      mask Display: disp('Pump')
  Subsystem7 : Subsystem
      mask Display: disp('Sensor\n y1')
  Subsystem8 : Subsystem
      mask Display: disp('TANK 2')
  Subsystem9 : Subsystem
      mask Display: disp('OPERATOR\nSET')
  mQp : Outport
  mUb : Outport  Port=2
  "Uo " : Outport  Port=3
  my1 : Outport  Port=4
  my2 : Outport  Port=5
  h1c : Outport  Port=6
  mUp : Outport  Port=7
  mq0 : Outport  Port=8
  y1 : Outport  Port=9
  vol1 : Outport  Port=10
  y2 : Outport  Port=11
  vol2 : Outport  Port=12
  mP1 : Outport  Port=13
  mP2 : Outport  Port=14
  wires:
  Subsystem12/1(mUb) -> mUb/1
  Subsystem3/1(Qv0) -> mq0/1, Subsystem10/2(mQo), Subsystem8/1(Qvo)
  Constant/1 -> Subsystem3/3(y0)
  Subsystem13/1(mUp) -> mUp/1
  Subsystem2/1(QVb) -> Subsystem8/2(Qvb), Subsystem1/2(Qvb)
  Subsystem11/1(mUp) -> Subsystem13/1(Up), Subsystem6/1(Up)
  Subsystem9/1(Out3) -> Subsystem11/1(h1c), h1c/1
  Subsystem9/2(Out1) -> "Uo "/1, Subsystem3/1(U0)
  Subsystem7/1(Out5) -> Subsystem11/2(my1), my1/1
  Subsystem14/1(mQp) -> mQp/1
  Subsystem4/1(Out5) -> Subsystem12/1(Ub), Subsystem2/1(Ub)
  Subsystem10/1(my2) -> Subsystem4/1(In2), my2/1
  Subsystem6/1(mUp) -> Subsystem1/1(Qp), Subsystem14/1(Qp)
  Subsystem7/2(Out1) -> y1/1
  Subsystem7/3(Out2) -> vol1/1
  Subsystem10/2(yy2) -> y2/1
  Subsystem10/3(vol2) -> vol2/1
  Subsystem5/1(mP1) -> mP1/1
  Subsystem1/1(y1) -> Subsystem5/1(y1), Subsystem2/2(y1), Subsystem7/1(In1)
  Subsystem15/1(mP2) -> mP2/1
  Subsystem8/1(y2) -> Subsystem3/2(y2), Subsystem15/1(y2), Subsystem2/3(y2), Subsystem10/1(y2)

== system CHEM_FULL_BENCHMARK/Long term T1 Water overflow PI/Process ==
  note: y2
  note: y1
  note: Ub
  note: Up
  note: Qvo
      | To users
  note: Qp
  note: Qvb
  Constant : Constant  Value=yo
  Subsystem1 : Subsystem
      mask Display: disp('TANK 1')
  Subsystem10 : Subsystem
      mask Display: disp('Sensor\n y2')
  Subsystem11 : Subsystem
      mask Display: disp('Controller 1')
  Subsystem12 : Subsystem
      mask Display: disp('Sensor\n Ub')
  Subsystem13 : Subsystem
      mask Display: disp('Sensor\n Up')
  Subsystem14 : Subsystem
      mask Display: disp('Sensor\n Qp')
  Subsystem15 : Subsystem
      mask Display: disp('Sensor\n P2')
  Subsystem2 : Subsystem
      mask Display: disp('Valve B')
  Subsystem3 : Subsystem
      mask Display: disp('Valve O')
  Subsystem4 : Subsystem
      mask Display: disp('Controller2')
  Subsystem5 : Subsystem
      mask Display: disp('Sensor\n P1')
  Subsystem6 : Subsystem
      mask Display: disp('Pump')
  Subsystem7 : Subsystem
      mask Display: disp('Sensor\n y1')
  Subsystem8 : Subsystem
      mask Display: disp('TANK 2')
  Subsystem9 : Subsystem
      mask Display: disp('OPERATOR\nSET')
  mQp : Outport
  mUb : Outport  Port=2
  "Uo " : Outport  Port=3
  my1 : Outport  Port=4
  my2 : Outport  Port=5
  h1c : Outport  Port=6
  mUp : Outport  Port=7
  mq0 : Outport  Port=8
  y1 : Outport  Port=9
  vol1 : Outport  Port=10
  y2 : Outport  Port=11
  vol2 : Outport  Port=12
  mP1 : Outport  Port=13
  mP2 : Outport  Port=14
  wires:
  Subsystem12/1(mUb) -> mUb/1
  Subsystem3/1(Qv0) -> mq0/1, Subsystem8/1(Qvo)
  Constant/1 -> Subsystem3/3(y0)
  Subsystem13/1(mUp) -> mUp/1
  Subsystem2/1(QVb) -> Subsystem8/2(Qvb), Subsystem1/2(Qvb)
  Subsystem11/1(mUp) -> Subsystem13/1(Up), Subsystem6/1(Up)
  Subsystem9/1(Out3) -> Subsystem11/1(h1c), h1c/1
  Subsystem9/2(Out1) -> "Uo "/1, Subsystem3/1(U0)
  Subsystem7/1(Out5) -> Subsystem11/2(my1), my1/1
  Subsystem14/1(mQp) -> mQp/1
  Subsystem4/1(Out5) -> Subsystem12/1(Ub), Subsystem2/1(Ub)
  Subsystem10/1(my2) -> my2/1, Subsystem4/1(In2)
  Subsystem6/1(mUp) -> Subsystem1/1(Qp), Subsystem14/1(Qp)
  Subsystem7/2(Out1) -> y1/1
  Subsystem7/3(Out2) -> vol1/1
  Subsystem10/2(yy2) -> y2/1
  Subsystem10/3(vol2) -> vol2/1
  Subsystem5/1(mP1) -> mP1/1
  Subsystem1/1(y1) -> Subsystem5/1(y1), Subsystem2/2(y1), Subsystem7/1(In1)
  Subsystem15/1(mP2) -> mP2/1
  Subsystem8/1(y2) -> Subsystem3/2(y2), Subsystem15/1(y2), Subsystem2/3(y2), Subsystem10/1(y2)

== system CHEM_FULL_BENCHMARK/Long term T1 Water overflow leak/Process ==
  note: y2
  note: y1
  note: Ub
  note: Up
  note: Qvo
      | To users
  note: Qp
  note: Qvb
  Constant : Constant  Value=yo
  Subsystem1 : Subsystem
      mask Display: disp('TANK 1')
  Subsystem10 : Subsystem
      mask Display: disp('Sensor\n y2')
  Subsystem11 : Subsystem
      mask Display: disp('Controller 1')
  Subsystem12 : Subsystem
      mask Display: disp('Sensor\n Ub')
  Subsystem13 : Subsystem
      mask Display: disp('Sensor\n Up')
  Subsystem14 : Subsystem
      mask Display: disp('Sensor\n Qp')
  Subsystem15 : Subsystem
      mask Display: disp('Sensor\n P2')
  Subsystem2 : Subsystem
      mask Display: disp('Valve B')
  Subsystem3 : Subsystem
      mask Display: disp('Valve O')
  Subsystem4 : Subsystem
      mask Display: disp('Controller2')
  Subsystem5 : Subsystem
      mask Display: disp('Sensor\n P1')
  Subsystem6 : Subsystem
      mask Display: disp('Pump')
  Subsystem7 : Subsystem
      mask Display: disp('Sensor\n y1')
  Subsystem8 : Subsystem
      mask Display: disp('TANK 2')
  Subsystem9 : Subsystem
      mask Display: disp('OPERATOR\nSET')
  mQp : Outport
  mUb : Outport  Port=2
  "Uo " : Outport  Port=3
  my1 : Outport  Port=4
  my2 : Outport  Port=5
  h1c : Outport  Port=6
  mUp : Outport  Port=7
  mq0 : Outport  Port=8
  y1 : Outport  Port=9
  vol1 : Outport  Port=10
  y2 : Outport  Port=11
  vol2 : Outport  Port=12
  mP1 : Outport  Port=13
  mP2 : Outport  Port=14
  wires:
  Subsystem12/1(mUb) -> mUb/1
  Subsystem3/1(Qv0) -> mq0/1, Subsystem8/1(Qvo)
  Constant/1 -> Subsystem3/3(y0)
  Subsystem13/1(mUp) -> mUp/1
  Subsystem2/1(QVb) -> Subsystem8/2(Qvb), Subsystem1/2(Qvb)
  Subsystem11/1(mUp) -> Subsystem13/1(Up), Subsystem6/1(Up)
  Subsystem9/1(Out3) -> Subsystem11/1(h1c), h1c/1
  Subsystem9/2(Out1) -> "Uo "/1, Subsystem3/1(U0)
  Subsystem7/1(Out5) -> Subsystem11/2(my1), my1/1
  Subsystem14/1(mQp) -> mQp/1
  Subsystem4/1(Out5) -> Subsystem12/1(Ub), Subsystem2/1(Ub)
  Subsystem10/1(my2) -> my2/1, Subsystem4/1(In2)
  Subsystem6/1(mUp) -> Subsystem1/1(Qp), Subsystem14/1(Qp)
  Subsystem7/2(Out1) -> y1/1
  Subsystem7/3(Out2) -> vol1/1
  Subsystem10/2(yy2) -> y2/1
  Subsystem10/3(vol2) -> vol2/1
  Subsystem5/1(mP1) -> mP1/1
  Subsystem1/1(y1) -> Subsystem5/1(y1), Subsystem2/2(y1), Subsystem7/1(In1)
  Subsystem15/1(mP2) -> mP2/1
  Subsystem8/1(y2) -> Subsystem3/2(y2), Subsystem15/1(y2), Subsystem2/3(y2), Subsystem10/1(y2)

== system CHEM_FULL_BENCHMARK/Reply attack/Process ==
  note: y2
  note: y1
  note: Ub
  note: Up
  note: Qvo
      | To users
  note: Qp
  note: Qvb
  Constant : Constant  Value=yo
  Subsystem1 : Subsystem
      mask Display: disp('TANK 1')
  Subsystem10 : Subsystem
      mask Display: disp('Sensor\n y2')
  Subsystem11 : Subsystem
      mask Display: disp('Controller 1')
  Subsystem12 : Subsystem
      mask Display: disp('Sensor\n Ub')
  Subsystem13 : Subsystem
      mask Display: disp('Sensor\n Up')
  Subsystem14 : Subsystem
      mask Display: disp('Sensor\n Qp')
  Subsystem15 : Subsystem
      mask Display: disp('Sensor\n P2')
  Subsystem2 : Subsystem
      mask Display: disp('Valve B')
  Subsystem3 : Subsystem
      mask Display: disp('Valve O')
  Subsystem4 : Subsystem
      mask Display: disp('Controller2')
  Subsystem5 : Subsystem
      mask Display: disp('Sensor\n P1')
  Subsystem6 : Subsystem
      mask Display: disp('Pump')
  Subsystem7 : Subsystem
      mask Display: disp('Sensor\n y1')
  Subsystem8 : Subsystem
      mask Display: disp('TANK 2')
  Subsystem9 : Subsystem
      mask Display: disp('OPERATOR\nSET')
  mQp : Outport
  mUb : Outport  Port=2
  "Uo " : Outport  Port=3
  my1 : Outport  Port=4
  my2 : Outport  Port=5
  h1c : Outport  Port=6
  mUp : Outport  Port=7
  mq0 : Outport  Port=8
  y1 : Outport  Port=9
  vol1 : Outport  Port=10
  y2 : Outport  Port=11
  vol2 : Outport  Port=12
  mP1 : Outport  Port=13
  mP2 : Outport  Port=14
  wires:
  Subsystem12/1(mUb) -> mUb/1
  Subsystem3/1(Qv0) -> mq0/1, Subsystem8/1(Qvo)
  Constant/1 -> Subsystem3/3(y0)
  Subsystem13/1(mUp) -> mUp/1
  Subsystem2/1(QVb) -> Subsystem8/2(Qvb), Subsystem1/2(Qvb)
  Subsystem11/1(mUp) -> Subsystem13/1(Up), Subsystem6/1(Up)
  Subsystem9/1(Out3) -> Subsystem11/1(h1c), h1c/1
  Subsystem9/2(Out1) -> "Uo "/1, Subsystem3/1(U0)
  Subsystem7/1(Out5) -> Subsystem11/2(my1), my1/1
  Subsystem14/1(mQp) -> mQp/1
  Subsystem4/1(Out5) -> Subsystem12/1(Ub), Subsystem2/1(Ub)
  Subsystem10/1(my2) -> my2/1, Subsystem4/1(In2)
  Subsystem6/1(mUp) -> Subsystem1/1(Qp), Subsystem14/1(Qp)
  Subsystem7/2(Out1) -> y1/1
  Subsystem7/3(Out2) -> vol1/1
  Subsystem10/2(yy2) -> y2/1
  Subsystem10/3(vol2) -> vol2/1
  Subsystem5/1(mP1) -> mP1/1
  Subsystem1/1(y1) -> Subsystem5/1(y1), Subsystem2/2(y1), Subsystem7/1(In1)
  Subsystem15/1(mP2) -> mP2/1
  Subsystem8/1(y2) -> Subsystem3/2(y2), Subsystem15/1(y2), Subsystem2/3(y2), Subsystem10/1(y2)

== system CHEM_FULL_BENCHMARK/T1 fault/Process ==
  note: y2
  note: y1
  note: Ub
  note: Up
  note: Qvo
      | To users
  note: Qp
  note: Qvb
  Constant : Constant  Value=yo
  Subsystem1 : Subsystem
      mask Display: disp('TANK 1')
  Subsystem10 : Subsystem
      mask Display: disp('Sensor\n y2')
  Subsystem11 : Subsystem
      mask Display: disp('Controller 1')
  Subsystem12 : Subsystem
      mask Display: disp('Sensor\n Ub')
  Subsystem13 : Subsystem
      mask Display: disp('Sensor\n Up')
  Subsystem14 : Subsystem
      mask Display: disp('Sensor\n Qp')
  Subsystem15 : Subsystem
      mask Display: disp('Sensor\n P2')
  Subsystem2 : Subsystem
      mask Display: disp('Valve B')
  Subsystem3 : Subsystem
      mask Display: disp('Valve O')
  Subsystem4 : Subsystem
      mask Display: disp('Controller2')
  Subsystem5 : Subsystem
      mask Display: disp('Sensor\n P1')
  Subsystem6 : Subsystem
      mask Display: disp('Pump')
  Subsystem7 : Subsystem
      mask Display: disp('Sensor\n y1')
  Subsystem8 : Subsystem
      mask Display: disp('TANK 2')
  Subsystem9 : Subsystem
      mask Display: disp('OPERATOR\nSET')
  mQp : Outport
  mUb : Outport  Port=2
  "Uo " : Outport  Port=3
  my1 : Outport  Port=4
  my2 : Outport  Port=5
  h1c : Outport  Port=6
  mUp : Outport  Port=7
  mq0 : Outport  Port=8
  y1 : Outport  Port=9
  vol1 : Outport  Port=10
  y2 : Outport  Port=11
  vol2 : Outport  Port=12
  mP1 : Outport  Port=13
  mP2 : Outport  Port=14
  wires:
  Subsystem12/1(mUb) -> mUb/1
  Subsystem3/1(Qv0) -> mq0/1, Subsystem8/1(Qvo)
  Constant/1 -> Subsystem3/3(y0)
  Subsystem13/1(mUp) -> mUp/1
  Subsystem2/1(QVb) -> Subsystem8/2(Qvb), Subsystem1/2(Qvb)
  Subsystem11/1(mUp) -> Subsystem13/1(Up), Subsystem6/1(Up)
  Subsystem9/1(Out3) -> Subsystem11/1(h1c), h1c/1
  Subsystem9/2(Out1) -> "Uo "/1, Subsystem3/1(U0)
  Subsystem7/1(Out5) -> Subsystem11/2(my1), my1/1
  Subsystem14/1(mQp) -> mQp/1
  Subsystem4/1(Out5) -> Subsystem12/1(Ub), Subsystem2/1(Ub)
  Subsystem10/1(my2) -> my2/1, Subsystem4/1(In2)
  Subsystem6/1(mUp) -> Subsystem1/1(Qp), Subsystem14/1(Qp)
  Subsystem7/2(Out1) -> y1/1
  Subsystem7/3(Out2) -> vol1/1
  Subsystem10/2(yy2) -> y2/1
  Subsystem10/3(vol2) -> vol2/1
  Subsystem5/1(mP1) -> mP1/1
  Subsystem1/1(y1) -> Subsystem5/1(y1), Subsystem2/2(y1), Subsystem7/1(In1)
  Subsystem15/1(mP2) -> mP2/1
  Subsystem8/1(y2) -> Subsystem3/2(y2), Subsystem15/1(y2), Subsystem2/3(y2), Subsystem10/1(y2)

== system CHEM_FULL_BENCHMARK/T1 hidden long theft/Process ==
  note: y2
  note: y1
  note: Ub
  note: Up
  note: Qvo
      | To users
  note: Qp
  note: Qvb
  Constant : Constant  Value=yo
  Subsystem1 : Subsystem
      mask Display: disp('TANK 1')
  Subsystem10 : Subsystem
      mask Display: disp('Sensor\n y2')
  Subsystem11 : Subsystem
      mask Display: disp('Controller 1')
  Subsystem12 : Subsystem
      mask Display: disp('Sensor\n Ub')
  Subsystem13 : Subsystem
      mask Display: disp('Sensor\n Up')
  Subsystem14 : Subsystem
      mask Display: disp('Sensor\n Qp')
  Subsystem15 : Subsystem
      mask Display: disp('Sensor\n P2')
  Subsystem2 : Subsystem
      mask Display: disp('Valve B')
  Subsystem3 : Subsystem
      mask Display: disp('Valve O')
  Subsystem4 : Subsystem
      mask Display: disp('Controller2')
  Subsystem5 : Subsystem
      mask Display: disp('Sensor\n P1')
  Subsystem6 : Subsystem
      mask Display: disp('Pump')
  Subsystem7 : Subsystem
      mask Display: disp('Sensor\n y1')
  Subsystem8 : Subsystem
      mask Display: disp('TANK 2')
  Subsystem9 : Subsystem
      mask Display: disp('OPERATOR\nSET')
  mQp : Outport
  mUb : Outport  Port=2
  "Uo " : Outport  Port=3
  my1 : Outport  Port=4
  my2 : Outport  Port=5
  h1c : Outport  Port=6
  mUp : Outport  Port=7
  mq0 : Outport  Port=8
  y1 : Outport  Port=9
  vol1 : Outport  Port=10
  y2 : Outport  Port=11
  vol2 : Outport  Port=12
  mP1 : Outport  Port=13
  mP2 : Outport  Port=14
  wires:
  Subsystem12/1(mUb) -> mUb/1
  Subsystem3/1(Qv0) -> mq0/1, Subsystem8/1(Qvo)
  Constant/1 -> Subsystem3/3(y0)
  Subsystem13/1(mUp) -> mUp/1
  Subsystem2/1(QVb) -> Subsystem8/2(Qvb), Subsystem1/2(Qvb)
  Subsystem11/1(mUp) -> Subsystem13/1(Up), Subsystem6/1(Up)
  Subsystem9/1(Out3) -> Subsystem11/1(h1c), h1c/1
  Subsystem9/2(Out1) -> "Uo "/1, Subsystem3/1(U0)
  Subsystem7/1(Out5) -> Subsystem11/2(my1), my1/1
  Subsystem14/1(mQp) -> mQp/1
  Subsystem4/1(Out5) -> Subsystem12/1(Ub), Subsystem2/1(Ub)
  Subsystem10/1(my2) -> my2/1, Subsystem4/1(In2)
  Subsystem6/1(mUp) -> Subsystem1/1(Qp), Subsystem14/1(Qp)
  Subsystem7/2(Out1) -> y1/1
  Subsystem7/3(Out2) -> vol1/1
  Subsystem10/2(yy2) -> y2/1
  Subsystem10/3(vol2) -> vol2/1
  Subsystem5/1(mP1) -> mP1/1
  Subsystem1/1(y1) -> Subsystem5/1(y1), Subsystem2/2(y1), Subsystem7/1(In1)
  Subsystem15/1(mP2) -> mP2/1
  Subsystem8/1(y2) -> Subsystem3/2(y2), Subsystem15/1(y2), Subsystem2/3(y2), Subsystem10/1(y2)

== system CHEM_FULL_BENCHMARK/T1 hidden short theft/Process ==
  note: y2
  note: y1
  note: Ub
  note: Up
  note: Qvo
      | To users
  note: Qp
  note: Qvb
  Constant : Constant  Value=yo
  Subsystem1 : Subsystem
      mask Display: disp('TANK 1')
  Subsystem10 : Subsystem
      mask Display: disp('Sensor\n y2')
  Subsystem11 : Subsystem
      mask Display: disp('Controller 1')
  Subsystem12 : Subsystem
      mask Display: disp('Sensor\n Ub')
  Subsystem13 : Subsystem
      mask Display: disp('Sensor\n Up')
  Subsystem14 : Subsystem
      mask Display: disp('Sensor\n Qp')
  Subsystem15 : Subsystem
      mask Display: disp('Sensor\n P2')
  Subsystem2 : Subsystem
      mask Display: disp('Valve B')
  Subsystem3 : Subsystem
      mask Display: disp('Valve O')
  Subsystem4 : Subsystem
      mask Display: disp('Controller2')
  Subsystem5 : Subsystem
      mask Display: disp('Sensor\n P1')
  Subsystem6 : Subsystem
      mask Display: disp('Pump')
  Subsystem7 : Subsystem
      mask Display: disp('Sensor\n y1')
  Subsystem8 : Subsystem
      mask Display: disp('TANK 2')
  Subsystem9 : Subsystem
      mask Display: disp('OPERATOR\nSET')
  mQp : Outport
  mUb : Outport  Port=2
  "Uo " : Outport  Port=3
  my1 : Outport  Port=4
  my2 : Outport  Port=5
  h1c : Outport  Port=6
  mUp : Outport  Port=7
  mq0 : Outport  Port=8
  y1 : Outport  Port=9
  vol1 : Outport  Port=10
  y2 : Outport  Port=11
  vol2 : Outport  Port=12
  mP1 : Outport  Port=13
  mP2 : Outport  Port=14
  wires:
  Subsystem12/1(mUb) -> mUb/1
  Subsystem3/1(Qv0) -> mq0/1, Subsystem8/1(Qvo)
  Constant/1 -> Subsystem3/3(y0)
  Subsystem13/1(mUp) -> mUp/1
  Subsystem2/1(QVb) -> Subsystem8/2(Qvb), Subsystem1/2(Qvb)
  Subsystem11/1(mUp) -> Subsystem13/1(Up), Subsystem6/1(Up)
  Subsystem9/1(Out3) -> Subsystem11/1(h1c), h1c/1
  Subsystem9/2(Out1) -> "Uo "/1, Subsystem3/1(U0)
  Subsystem7/1(Out5) -> Subsystem11/2(my1), my1/1
  Subsystem14/1(mQp) -> mQp/1
  Subsystem4/1(Out5) -> Subsystem12/1(Ub), Subsystem2/1(Ub)
  Subsystem10/1(my2) -> my2/1, Subsystem4/1(In2)
  Subsystem6/1(mUp) -> Subsystem1/1(Qp), Subsystem14/1(Qp)
  Subsystem7/2(Out1) -> y1/1
  Subsystem7/3(Out2) -> vol1/1
  Subsystem10/2(yy2) -> y2/1
  Subsystem10/3(vol2) -> vol2/1
  Subsystem5/1(mP1) -> mP1/1
  Subsystem1/1(y1) -> Subsystem5/1(y1), Subsystem2/2(y1), Subsystem7/1(In1)
  Subsystem15/1(mP2) -> mP2/1
  Subsystem8/1(y2) -> Subsystem3/2(y2), Subsystem15/1(y2), Subsystem2/3(y2), Subsystem10/1(y2)

== system CHEM_FULL_BENCHMARK/T1 semi hidden long theft/Process ==
  note: y2
  note: y1
  note: Ub
  note: Up
  note: Qvo
      | To users
  note: Qp
  note: Qvb
  Constant : Constant  Value=yo
  Subsystem1 : Subsystem
      mask Display: disp('TANK 1')
  Subsystem10 : Subsystem
      mask Display: disp('Sensor\n y2')
  Subsystem11 : Subsystem
      mask Display: disp('Controller 1')
  Subsystem12 : Subsystem
      mask Display: disp('Sensor\n Ub')
  Subsystem13 : Subsystem
      mask Display: disp('Sensor\n Up')
  Subsystem14 : Subsystem
      mask Display: disp('Sensor\n Qp')
  Subsystem15 : Subsystem
      mask Display: disp('Sensor\n P2')
  Subsystem2 : Subsystem
      mask Display: disp('Valve B')
  Subsystem3 : Subsystem
      mask Display: disp('Valve O')
  Subsystem4 : Subsystem
      mask Display: disp('Controller2')
  Subsystem5 : Subsystem
      mask Display: disp('Sensor\n P1')
  Subsystem6 : Subsystem
      mask Display: disp('Pump')
  Subsystem7 : Subsystem
      mask Display: disp('Sensor\n y1')
  Subsystem8 : Subsystem
      mask Display: disp('TANK 2')
  Subsystem9 : Subsystem
      mask Display: disp('OPERATOR\nSET')
  mQp : Outport
  mUb : Outport  Port=2
  "Uo " : Outport  Port=3
  my1 : Outport  Port=4
  my2 : Outport  Port=5
  h1c : Outport  Port=6
  mUp : Outport  Port=7
  mq0 : Outport  Port=8
  y1 : Outport  Port=9
  vol1 : Outport  Port=10
  y2 : Outport  Port=11
  vol2 : Outport  Port=12
  mP1 : Outport  Port=13
  mP2 : Outport  Port=14
  wires:
  Subsystem12/1(mUb) -> mUb/1
  Subsystem3/1(Qv0) -> mq0/1, Subsystem8/1(Qvo)
  Constant/1 -> Subsystem3/3(y0)
  Subsystem13/1(mUp) -> mUp/1
  Subsystem2/1(QVb) -> Subsystem8/2(Qvb), Subsystem1/2(Qvb)
  Subsystem11/1(mUp) -> Subsystem13/1(Up), Subsystem6/1(Up)
  Subsystem9/1(Out3) -> Subsystem11/1(h1c), h1c/1
  Subsystem9/2(Out1) -> "Uo "/1, Subsystem3/1(U0)
  Subsystem7/1(Out5) -> my1/1, Subsystem11/2(my1)
  Subsystem14/1(mQp) -> mQp/1
  Subsystem4/1(Out5) -> Subsystem12/1(Ub), Subsystem2/1(Ub)
  Subsystem10/1(my2) -> my2/1, Subsystem4/1(In2)
  Subsystem6/1(mUp) -> Subsystem1/1(Qp), Subsystem14/1(Qp)
  Subsystem7/2(Out1) -> y1/1
  Subsystem7/3(Out2) -> vol1/1
  Subsystem10/2(yy2) -> y2/1
  Subsystem10/3(vol2) -> vol2/1
  Subsystem5/1(mP1) -> mP1/1
  Subsystem1/1(y1) -> Subsystem2/2(y1), Subsystem5/1(y1), Subsystem7/1(In1)
  Subsystem15/1(mP2) -> mP2/1
  Subsystem8/1(y2) -> Subsystem3/2(y2), Subsystem15/1(y2), Subsystem2/3(y2), Subsystem10/1(y2)

== system CHEM_FULL_BENCHMARK/T1 short theft/Process ==
  note: y2
  note: y1
  note: Ub
  note: Up
  note: Qvo
      | To users
  note: Qp
  note: Qvb
  Constant : Constant  Value=yo
  Subsystem1 : Subsystem
      mask Display: disp('TANK 1')
  Subsystem10 : Subsystem
      mask Display: disp('Sensor\n y2')
  Subsystem11 : Subsystem
      mask Display: disp('Controller 1')
  Subsystem12 : Subsystem
      mask Display: disp('Sensor\n Ub')
  Subsystem13 : Subsystem
      mask Display: disp('Sensor\n Up')
  Subsystem14 : Subsystem
      mask Display: disp('Sensor\n Qp')
  Subsystem15 : Subsystem
      mask Display: disp('Sensor\n P2')
  Subsystem2 : Subsystem
      mask Display: disp('Valve B')
  Subsystem3 : Subsystem
      mask Display: disp('Valve O')
  Subsystem4 : Subsystem
      mask Display: disp('Controller2')
  Subsystem5 : Subsystem
      mask Display: disp('Sensor\n P1')
  Subsystem6 : Subsystem
      mask Display: disp('Pump')
  Subsystem7 : Subsystem
      mask Display: disp('Sensor\n y1')
  Subsystem8 : Subsystem
      mask Display: disp('TANK 2')
  Subsystem9 : Subsystem
      mask Display: disp('OPERATOR\nSET')
  mQp : Outport
  mUb : Outport  Port=2
  "Uo " : Outport  Port=3
  my1 : Outport  Port=4
  my2 : Outport  Port=5
  h1c : Outport  Port=6
  mUp : Outport  Port=7
  mq0 : Outport  Port=8
  y1 : Outport  Port=9
  vol1 : Outport  Port=10
  y2 : Outport  Port=11
  vol2 : Outport  Port=12
  mP1 : Outport  Port=13
  mP2 : Outport  Port=14
  wires:
  Subsystem12/1(mUb) -> mUb/1
  Subsystem3/1(Qv0) -> mq0/1, Subsystem8/1(Qvo)
  Constant/1 -> Subsystem3/3(y0)
  Subsystem13/1(mUp) -> mUp/1
  Subsystem2/1(QVb) -> Subsystem8/2(Qvb), Subsystem1/2(Qvb)
  Subsystem11/1(mUp) -> Subsystem13/1(Up), Subsystem6/1(Up)
  Subsystem9/1(Out3) -> Subsystem11/1(h1c), h1c/1
  Subsystem9/2(Out1) -> "Uo "/1, Subsystem3/1(U0)
  Subsystem7/1(Out5) -> Subsystem11/2(my1), my1/1
  Subsystem14/1(mQp) -> mQp/1
  Subsystem4/1(Out5) -> Subsystem12/1(Ub), Subsystem2/1(Ub)
  Subsystem10/1(my2) -> my2/1, Subsystem4/1(In2)
  Subsystem6/1(mUp) -> Subsystem1/1(Qp), Subsystem14/1(Qp)
  Subsystem7/2(Out1) -> y1/1
  Subsystem7/3(Out2) -> vol1/1
  Subsystem10/2(yy2) -> y2/1
  Subsystem10/3(vol2) -> vol2/1
  Subsystem5/1(mP1) -> mP1/1
  Subsystem1/1(y1) -> Subsystem5/1(y1), Subsystem2/2(y1), Subsystem7/1(In1)
  Subsystem15/1(mP2) -> mP2/1
  Subsystem8/1(y2) -> Subsystem3/2(y2), Subsystem15/1(y2), Subsystem2/3(y2), Subsystem10/1(y2)
